simulink model "HevMmReferenceApplication"  (R2021b)
settings: Solver=ode23tb  StartTime=0  StopTime=1800  RelTol=1e-3  EnableMultiTasking=on
model workspace (MAT data in the model file):
  Active_Scenario_Index = 1
  BattChrgMax = -105500
  BattDischrgMax = 211000
  BattTempInit = 25
  Battery.SOC_LUT = [0.01 0.02 0.03 0.04 0.05 0.06 0.07 0.08 0.09 0.1 0.11 0.12 0.13 0.14 0.15 0.16 0.17 0.18 0.19 0.2 0.21 0.22 0.23 0.24 0.25 0.26 0.27 0.28 0.29 0.3 0.31 0.32 0.33 0.34 0.35 0.36 0.37 0.38 0.39 0.4 0.41 0.42 0.43 0.44 0.45 0.46 0.47 0.48 0.49 0.5 0.51 0.52 0.53 0.54 0.55 0.56 0.57 0.58 0.59 0.6 0.61 0.62 0.63 0.64 0.65 0.66 0.67 0.68 0.69 0.7 0.71 0.72 0.73 0.74 0.75 0.76 0.77 0.78 0.79 0.8 0.81 0.82 0.83 0.84 0.85 0.86 0.87 0.88 0.89 0.9 0.91 0.92 0.93 0.94 0.95 0.96 0.97 0.98 0.99 1]
  Battery.Temperature_LUT = [-10 0 25 40]
  Battery.Capacity_LUT = [4.04528301887 4.19622641509 4.8 4.73962264151]
  Battery.Em_LUT = [2.67308083891 2.74411674384 2.80408613071 2.86247711994 2.90851059763 2.94904306488 2.9829846776 3.01467102589 3.04031502638 3.06256828113 3.08180972392 3.09994219643 ... (400 elements, 100x4)]
  Battery.R0_LUT = [0.0569026752707 0.0575506938969 0.0576730924021 0.0575627404981 0.0573787336615 0.0571931123197 0.0568199985482 0.056411926464 0.0561974340667 0.0560805640861 0.0557640899305 0.055275807865 ... (400 elements, 100x4)]
  Battery.R1_LUT = [0.0035 0.0035 0.0035 0.0035 0.0035 0.0035 0.0035 0.0035 0.0035 0.0035 0.0035 0.0035 ... (400 elements, 100x4)]
  Battery.C1_LUT = [5000 5000 5000 5000 5000 5000 5000 5000 5000 5000 5000 5000 ... (400 elements, 100x4)]
  Battery.Mass = 0.047
  Battery.ThermalMass = 44
  Battery.R_bleed = 20
  Battery.h_conv = 5
  Battery.cell_area = 0.0037
  Battery.TempInit = 25
  Battery.SOCInit = 0.75
  Battery.Model = 'panasonic ncr18650bd'
  Battery.DischargeCycle_LUT = [1 5 9 13 17 21 25 29 33 37 41 45 49 53 57 61 65 69 73 77 81 85 89 93 97 101 105 109 113 117 121 125 129 133 137 141 145 149 153 157 161 165 169 173 177 181 185 189 193 197 201 205 209 213 217 221 225 229 233 237 241 245 249 253 257 261 265 269 273 277 281 285 289 293 297 301 305 309 313 317]
  Battery.deltaEm_LUT = [0 -0.363115641304 -0.600096647258 -0.689070000839 -0.76773380251 -0.846397604181 -0.926368385458 -0.992711297521 -1.05704974111 -1.12227693902 -1.19018070587 -1.25808447272 -1.31699459748 -1.35876443799 -1.40168267642 -1.44460091485 -1.48751915327 -1.5304373917 -1.57335563013 -1.62198241593 -1.67232184498 -1.71858340023 -1.76179802551 -1.8050126508 -1.84822727608 -1.8917937136 -1.93575272784 -1.97971174208 -2.02367075632 -2.06762977056 -2.11171979109 -2.15588700406 -2.19980020032 -2.24365853098 -2.28751686164 -2.33137519231 -2.37523352297 -2.41909185363 -2.45982559031 -2.49599372373 -2.53216185715 -2.56832999058 -2.604498124 -2.64066625743 -2.67683439085 -2.71300252428 -2.7491706577 -2.78367585394 -2.81632179346 -2.8483348579 -2.88034792233 -2.91236098677 -2.94437405121 -2.97638711564 -3.00840018008 -3.04041324451 -3.07260346059 -3.10359008254 -3.13082308991 -3.15805609728 -3.18528910464 -3.21252211201 -3.23975511938 -3.26698812675 -3.29422113412 -3.32122400938 -3.3463475604 -3.37152613073 -3.39670470105 -3.42188327138 -3.4470618417 -3.47224041203 -3.49938358795 -3.52900276724 -3.55862194653 -3.58824112582 -3.6178603051 -3.64748858268 -3.67711690909 -3.70674523549]
  Battery.deltaCapacity_LUT = [0 -0.860019120059 -1.71332421702 -2.0819400264 -2.45055583577 -2.81917164515 -3.18778745452 -3.48884924257 -3.7808148236 -4.07278040463 -4.36474598566 -4.6567115667 -4.91000721732 -5.08494410056 -5.2598809838 -5.43481786703 -5.60975475027 -5.78469163351 -5.95962851674 -6.13456539998 -6.30950228322 -6.47026795816 -6.62044510558 -6.77062225299 -6.92079940041 -7.07097654783 -7.22115369524 -7.37133084266 -7.52150799007 -7.67168513749 -7.82230984162 -7.97319825819 -8.12408667477 -8.27497509134 -8.42586350792 -8.57675192449 -8.72764034107 -8.87852875764 -9.01789522921 -9.13717923376 -9.25646323831 -9.37574724285 -9.4950312474 -9.61431525195 -9.73359925649 -9.85288326104 -9.97216726558 -10.0914512701 -10.2059878191 -10.3183039593 -10.4306200996 -10.5429362398 -10.65525238 -10.7675685203 -10.8798846605 -10.9922008008 -11.104516941 -11.2125891929 -11.3075699376 -11.4025506823 -11.4975314271 -11.5925121718 -11.6874929166 -11.7824736613 -11.877454406 -11.9716325175 -12.0588579537 -12.1460833899 -12.2333088261 -12.3205342623 -12.4077596986 -12.4949851348 -12.5890165008 -12.6916254178 -12.7942343349 -12.8968432519 -12.999452169 -13.102061086 -13.2046700031 -13.3072789201]
  Battery.cond_thickness = 0.001
  Battery.thermal_conductivity = 205
  BrkPrsMax = 5000000
  CellType = 1
  ChrgLmt_bpt = [1 1 1 1 1 1 1 1 0.7 0.35 0]
  DischrgLmt_bpt = [0 0.35 0.7 1 1 1 1 1 1 1 1]
  MotMapEff = 0
  MotSpd = [0 1600 3200 4477.56 4800 6400 8000 9600 11200 12800 14400 16000]
  MotTrq = [450 450 450 450 419.771162405 314.828371804 251.862697443 209.885581202 179.901926745 157.414185902 139.923720802 125.931348721]
  Ndiff = 9.04
  Np_Module = 31
  Ns_Module = 24
  NumModules = 4
  OverCellVoltageLimit = 4.19999980927
  RegenBrkCutOff = [0 1]
  RegenBrkSpd_bpt = [5 9]
  Rm = 0.15
  SOC_bpt = [0 10 20 30 40 50 60 70 80 90 100]
  T_eff_bp = [0 32.1428571429 64.2857142857 96.4285714286 128.571428571 160.714285714 192.857142857 225 257.142857143 289.285714286 321.428571429 353.571428571 385.714285714 417.857142857 450]
  TestCase = 1
  UnderCellVoltageLimit = 2.5
  disk_abore = 0.05
  efficiency_table = [86.7  86.7  86.7  86.7  86.7  86.7  86.7  86.7  86.7  86.7  86.7  86.7  86.7  86.7  86.7; 86.7  86.7  86.7  86.7  86.7  86.7  86.7  86.7  86.7  86.7  86.7  86.7  86.7  86.7  86.7; 86.7  86.7  91.8  91.8  91.8  91.8  91.8  91.8  91.8  91.8  89.76  89.76  89.76  89.76  89.76; 86.7  86.7  93.84  93.84  93.84  93.84  93.84  93.84  93.84  93.84  93.84  91.8  91.8  91.8  91.8; 86.7  86.7  93.84  93.84  94.86  94.86  94.86  94.86  93.84  93.84  93.84  91.8  91.8  91.8  91.8; 86.7  86.7  94.86  95.88  95.88  95.88  95.88  95.88  95.88  95.88  95.88  95.88  95.88  95.88  95.88; 86.7  86.7  94.86  95.88  95.88  96.9  96.9  96.9  96.9  96.9  96.9  96.9  96.9  96.9  96.9; 86.7  86.7  94.86  95.88  95.88  96.9  96.9  96.9  96.9  96.9  96.9  96.9  96.9  96.9  96.9; 86.7  86.7  94.86  95.88  96.9  96.9  96.9  96.9  96.9  96.9  96.9  96.9  96.9  96.9  96.9; 86.7  86.7  94.86  95.88  96.9  96.9  96.9  96.9  96.9  96.9  96.9  96.9  96.9  96.9  96.9; 86.7  86.7  94.86  95.88  95.88  95.88  95.88  95.88  95.88  95.88  95.88  95.88  95.88  95.88  95.88; 86.7  86.7  91.8  93.84  94.86  94.86  94.86  94.86  94.86  94.86  94.86  94.86  94.86  94.86  94.86]
  mu_kinetic = 0.35
  num_pads = 2
  ts = 0.1
  w_eff_bp = [0 1600 3200 4477.56 4800 6400 8000 9600 11200 12800 14400 16000]
undefined symbols (not defined in the file or in its folder): sigbuilder_block, SRE
libraries: autolibsharedcommon x4, autolibshared x3, simulink x1, slpidlib x1
(part 1 of 2)
settings Model: DataDictionary=HevMmReferenceApplication.sldd  ModifiedByFormat=The MathWorks, Inc.  SimulationMode=accelerator  PauseTimes=23.46  Creator=The MathWorks, Inc.  LastModifiedBy=The MathWorks, Inc.
settings SolverCC: SolverJacobianMethodControl=FullPerturbation  ZeroCrossAlgorithm=Adaptive  AlgebraicLoopSolver=TrustRegion  MinimalZcImpactIntegration=on
settings DataIOCC: DSMLogging=off  ReturnWorkspaceOutputs=off
settings DebuggingCC: UnderspecifiedInitializationDetection=Classic  MergeDetectMultiDrivingBlocksExec=none  MaskedZcDiagnostic=none  IgnoredZcDiagnostic=none  ParameterPrecisionLossMsg=none  ModelReferenceExtraNoncontSigs=none  PregeneratedLibrarySubsystemCodeDiagnostic=none  SFMachineParentedDataDiag=warning  ArithmeticOperatorsInVariantConditions=warning
settings ModelReferenceCC: UpdateModelReferenceTargets=IfOutOfDate  ModelReferenceMinAlgLoopOccurrences=on  PropagateSignalLabelsOutOfModel=off
settings SFSimCC: SimUseLocalCustomCode=off
settings RTWCC: RTWUseLocalCustomCode=off
settings CodeAppCC: StateflowObjectComments=on
settings GRTTargetCC: TargetLangStandard=C89/C90 (ANSI)
settings ConfigComp: CovMetricSettings=dsw  CovSaveCumulativeToWorkspaceVar=on  CovSaveSingleToWorkspaceVar=on  CovExternalEMLEnable=off

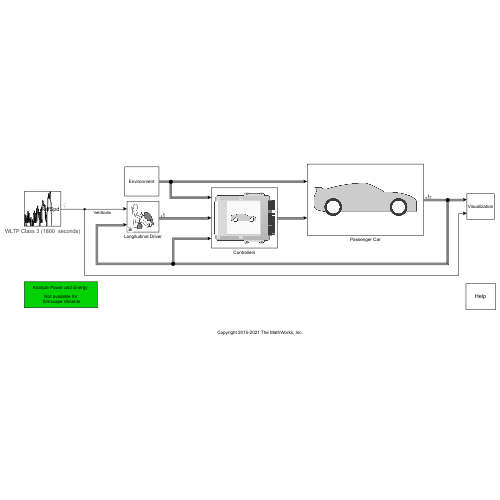
[thumbnail: Simulink's stored preview of the top-level diagram]
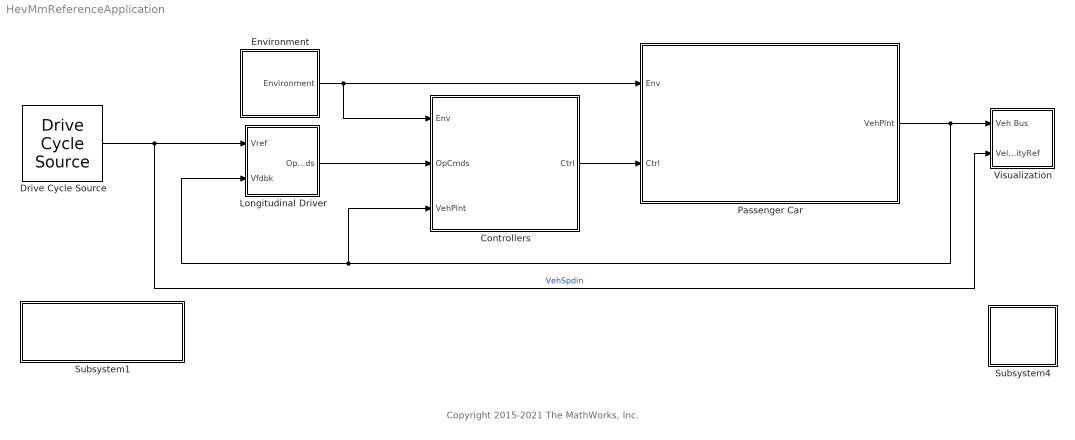
== system HevMmReferenceApplication ==
  note: Copyright 2015-2021 The MathWorks, Inc.
  Controllers : Subsystem
      mask Display: image('SystemControllers.png', 'center')
  Drive Cycle Source : autolibshared/Drive Cycle Source  cycleVar=WLTP Class 3  fileVar=L:\Bauto\matlab\test\toolbox\shared\autoblks\scenario\adac.txt  tfinal="1800  seconds"  cycleRepeat=off  outAccPort=off  outGearPort=off  gearList=No gear data  t_wot1=1  xdot_woto=0  xdot_wot1=10  t_wot2=199  xdot_wot2=0  t_wotend=200  srcUnit=m/s  outUnit=m/s  srcAccUnit=m/s/s  outAccUnit=m/s^2  dt=0  aMode=1  faultOption=off  velBnd=2  velBndUnit=mph  inUnit=m/s  timeBnd=1  failOption=off  stopSim=off  maxFaultCnt=10  maxFaultTime=2  maxTotFaultTime=15  traceOption=off  dtTrace=1  traceWindow=10  lastDCname=WLTP Class 3  lastOutUnit=mph  lastDT=0  lastTB=1  lastSB=2  forceCalcBound=off
      settings: SourceProductBaseCode=PW,DR,MT,UV,VE
  Environment : Subsystem
      mask Display: disp(getString(message('autoblks:autoblkVehMask:environ')))
  Longitudinal Driver : Subsystem  Variant=on  VariantControlMode=label  VariantControl=Variant1  LabelModeActiveChoice=2
      mask Display:
      | if strcmp('1',get_param(gcb,'ActiveVariant'))
      |     disp('Open Loop')
      | else
      |     image('LongitudinalDriver.png','center');
      | end
  Passenger Car : Subsystem
      mask Display: image('PassengerVehicle.png', 'center')
  Subsystem1 : Subsystem
      settings: OpenFcn=edit GenerateEnergyReport
      mask Display: disp(getString(message('autoblks:autoblkVehMask:powAndEne')))
  Subsystem4 : Subsystem
      settings: OpenFcn=helpview([docroot,'/toolbox/autoblks/helptargets.map'], 'hybrid_refapp')
      mask Display: disp(getString(message('autoblks:autoblkVehMask:help')))
  Visualization : Subsystem
      mask Display: disp(getString(message('autoblks:autoblkVehMask:visual')))
  wires:
  Longitudinal Driver/1(" OpCmds") -> Controllers/2(OpCmds)
  Drive Cycle Source/1 -> Longitudinal Driver/1("Vref "), Visualization/2(VelocityRef)  "VehSpdin"
  Environment/1(Environment) -> Passenger Car/1(Env), Controllers/1(Env)
  Controllers/1(Ctrl) -> Passenger Car/2(Ctrl)
  Passenger Car/1(VehPlnt) -> Longitudinal Driver/2("Vfdbk "), Controllers/3(VehPlnt), Visualization/1(Veh Bus)

== system HevMmReferenceApplication/Controllers ==
  Env : Inport
  OpCmds : Inport  Port=2
  VehPlnt : Inport  Port=3
  Bus Creator : BusCreator  Inputs=2
  PCM Input : Subsystem
  PCM Output : Subsystem
  Powertrain Control Module (PCM) : Subsystem
  Ctrl : Outport  VectorParamsAs1DForOutWhenUnconnected=off
  wires:
  PCM Output/1(EngCtrl) -> [EngCtrl]
  Bus Creator/1 -> Ctrl/1
  [EngCtrl] -> Bus Creator/1
  [PtCtrl] -> Bus Creator/2
  Env/1 -> [Environment]
  [OpCmds] -> PCM Input/4(OpCmds)
  VehPlnt/1 -> [VehPlnt]
  OpCmds/1 -> [OpCmds]
  [PtCtrl] -> PCM Input/1(PtCtrl)
  [Environment] -> PCM Input/2(Env)
  [VehPlnt] -> PCM Input/3(VehPlnt)
  PCM Output/2(PtCtrl) -> [PtCtrl]
  PCM Input/1(TrqCmd) -> Powertrain Control Module (PCM)/1(TrqCmd)
  PCM Input/2(EngSpd) -> Powertrain Control Module (PCM)/2(EngSpd)
  PCM Input/3(Map) -> Powertrain Control Module (PCM)/3(Map)
  PCM Input/4(Mat) -> Powertrain Control Module (PCM)/4(Mat)
  PCM Input/5(ThrPosPct) -> Powertrain Control Module (PCM)/5(ThrPosPct)
  PCM Input/6(WgAreaPct) -> Powertrain Control Module (PCM)/6(WgAreaPct)
  PCM Input/7(IntkCamPhase) -> Powertrain Control Module (PCM)/7(IntkCamPhase)
  PCM Input/8(ExhCamPhase) -> Powertrain Control Module (PCM)/8(ExhCamPhase)
  PCM Input/9(TurboRackPos) -> Powertrain Control Module (PCM)/9(TurboRackPos)
  PCM Input/10(EgrVlvAreaPct) -> Powertrain Control Module (PCM)/10(EgrVlvAreaPct)
  PCM Input/11(VarCompRatioPos) -> Powertrain Control Module (PCM)/11(VarCompRatioPos)
  PCM Input/12(IntkVlvLift) -> Powertrain Control Module (PCM)/12(IntkVlvLift)
  PCM Input/13(VarIntkRunLen) -> Powertrain Control Module (PCM)/13(VarIntkRunLen)
  PCM Input/14(Afr) -> Powertrain Control Module (PCM)/14(Afr)
  PCM Input/15(IntkSwirlVlvPos) -> Powertrain Control Module (PCM)/15(IntkSwirlVlvPos)
  PCM Input/16(TurboSpd) -> Powertrain Control Module (PCM)/16(TurboSpd)
  PCM Input/17(AmbPrs) -> Powertrain Control Module (PCM)/17(AmbPrs)
  PCM Input/18(AccCmd) -> Powertrain Control Module (PCM)/18(AccCmd)
  PCM Input/19(DecCmd) -> Powertrain Control Module (PCM)/19(DecCmd)
  PCM Input/25(VehSpdFdbk) -> Powertrain Control Module (PCM)/25(VehSpdFdbk)
  PCM Input/26(EngSpdFdbk) -> Powertrain Control Module (PCM)/26(EngSpdFdbk)
  PCM Input/27(EngCltchState) -> Powertrain Control Module (PCM)/27(EngCltchState)
  PCM Input/28(BattSoc) -> Powertrain Control Module (PCM)/28(BattSoc)
  PCM Input/29(BattPwr) -> Powertrain Control Module (PCM)/29(BattPwr)
  PCM Input/30(BattCrnt) -> Powertrain Control Module (PCM)/30(BattCrnt)
  PCM Input/31(EngCltchOutSpd) -> Powertrain Control Module (PCM)/31(EngCltchOutSpd)
  PCM Input/32(MotSpd) -> Powertrain Control Module (PCM)/32(MotSpd)
  PCM Input/33(GenPwrElec) -> Powertrain Control Module (PCM)/33(GenPwrElec)
  PCM Input/34(GenPwrMech) -> Powertrain Control Module (PCM)/34(GenPwrMech)
  PCM Input/20(IgSw) -> Powertrain Control Module (PCM)/20(IgSw)
  PCM Input/22(Ect) -> Powertrain Control Module (PCM)/22(Ect)
  PCM Input/23(EgrDeltaPrs) -> Powertrain Control Module (PCM)/23(EgrVlvDeltaPrs)
  PCM Input/24(EgrInTemp) -> Powertrain Control Module (PCM)/24(EgrVlvInTemp)
  PCM Input/21(Iat) -> Powertrain Control Module (PCM)/21(Iat)
  Powertrain Control Module (PCM)/1(ThrPosPctCmd) -> PCM Output/1(ThrPosPctCmd)
  Powertrain Control Module (PCM)/2(WgAreaPctCmd) -> PCM Output/2(WgAreaPctCmd)
  Powertrain Control Module (PCM)/3(InjPw) -> PCM Output/3(InjPw)
  Powertrain Control Module (PCM)/4(FuelMainSoi) -> PCM Output/4(FuelMainSoi)
  Powertrain Control Module (PCM)/5(SpdAdv) -> PCM Output/5(SpkAdv)
  Powertrain Control Module (PCM)/6(IntkCamPhaseCmd) -> PCM Output/6(IntkCamPhaseCmd)
  Powertrain Control Module (PCM)/7(ExhCamPhaseCmd) -> PCM Output/7(ExhCamPhaseCmd)
  Powertrain Control Module (PCM)/8(TurboRackPosCmd) -> PCM Output/8(TurboRackPosCmd)
  Powertrain Control Module (PCM)/9(EgrVlvAreaPctCmd) -> PCM Output/9(EgrVlvAreaPctCmd)
  Powertrain Control Module (PCM)/10(VarCompRatioPosCmd) -> PCM Output/10(VarCompRatioPosCmd)
  Powertrain Control Module (PCM)/11(IntkVlvLiftCmd) -> PCM Output/11(IntkVlvLiftCmd)
  Powertrain Control Module (PCM)/12(VarIntkRunLenCmd) -> PCM Output/12(VarIntkRunLenCmd)
  Powertrain Control Module (PCM)/13(ClsdLpFuelMult) -> PCM Output/13(ClsdLpFuelMult)
  Powertrain Control Module (PCM)/14(IntkSwirlVlvPosCmd) -> PCM Output/14(IntkSwirlVlvPosCmd)
  Powertrain Control Module (PCM)/15(TrqCmdISC) -> PCM Output/15(TrqCmdISC)
  Powertrain Control Module (PCM)/16(LoadCmd) -> PCM Output/16(LoadCmd)
  Powertrain Control Module (PCM)/17(EstIntkPortFlw) -> PCM Output/17(EstIntkPortFlw)
  Powertrain Control Module (PCM)/18(EngCltchCmd) -> PCM Output/18(EngCltchCmd)
  Powertrain Control Module (PCM)/19(EngTrqCmd) -> PCM Output/19(EngineTrqCmd)
  Powertrain Control Module (PCM)/20(GenTrqCmd) -> PCM Output/20(GenTrqCmd)
  Powertrain Control Module (PCM)/21(MotTrqCmd) -> PCM Output/21(MotTrqCmd)
  Powertrain Control Module (PCM)/22(BrakeCmd) -> PCM Output/22(BrakeCmd)
  PCM Input/35(BMS_Sensors) -> Powertrain Control Module (PCM)/35(BMS_Sensors)
  Powertrain Control Module (PCM)/23(BMS_Info) -> PCM Output/23(BMS_Info)
  Powertrain Control Module (PCM)/24(BMS_Cmd) -> PCM Output/24(BMS_Cmd)

== system HevMmReferenceApplication/Environment ==
  Bus Creator : BusCreator  Inputs=4
  Bus Creator3 : BusCreator  Inputs=3
  Bus Creator4 : BusCreator  Inputs=2
  Bus Creator5 : BusCreator  Inputs=2
  Constant2 : Constant  Value=0
  Constant3 : Constant  Value=0
  Constant6 : Constant  Value=300
  Constant7 : Constant  Value=101325
  Ground{,1..3} (4 alike) : Ground
  Environment : Outport  VectorParamsAs1DForOutWhenUnconnected=off
  wires:
  Ground2/1 -> Bus Creator5/1  "lam_mu_x"
  Ground3/1 -> Bus Creator5/2  "lam_mu_y"
  Bus Creator5/1 -> Bus Creator4/2  "Ground_mu"
  Bus Creator4/1 -> Bus Creator/3  "Ground"
  Bus Creator3/1 -> Bus Creator/4  "Wind"
  Constant3/1 -> Bus Creator3/1  "wind_x"
  Ground/1 -> Bus Creator3/2  "wind_y"
  Ground1/1 -> Bus Creator3/3  "wind_z"
  Constant6/1 -> Bus Creator/1  "Temp"
  Constant2/1 -> Bus Creator4/1  "Grade"
  Bus Creator/1 -> Environment/1  "Environment"
  Constant7/1 -> Bus Creator/2  "Baro"

== system HevMmReferenceApplication/Longitudinal Driver ==
  note: To switch variants, right-click on this subsystem (from one level above) and chose:
      | Variant, Active choice, <your selection>
  "Vref " : Inport
  "Vfdbk " : Inport  Port=2
  Longitudinal Driver : Subsystem  VariantControl=0
      mask Display: image('LongitudinalDriver.png', 'center')
  Open Loop : Subsystem  VariantControl=1
      mask Display: disp('Open Loop')
  PID : Subsystem  TreatAsAtomicUnit=on  VariantControl=2
  " OpCmds" : Outport  VectorParamsAs1DForOutWhenUnconnected=off

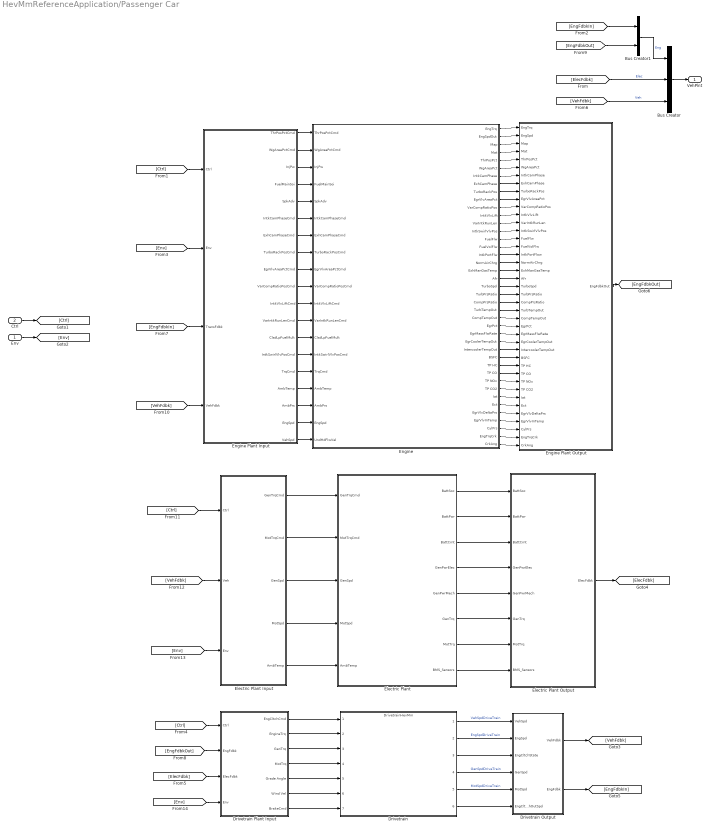
== system HevMmReferenceApplication/Passenger Car ==
  Env : Inport
  Ctrl : Inport  Port=2
  Bus Creator : BusCreator  Inputs=3
  Bus Creator1 : BusCreator  Inputs=2
  Drivetrain : ModelReference  ModelNameDialog=DrivetrainHevMm.slx  SimulationMode=Normal  ModelReferenceVersion=5.24
  Drivetrain Output : Subsystem
  Drivetrain Plant Input : Subsystem
  Electric Plant : Subsystem
  Electric Plant Input : Subsystem
  Electric Plant Output : Subsystem
  Engine : Subsystem  Variant=on  VariantControlMode=label  LabelModeActiveChoice=SiMappedEngine
  Engine Plant Input : Subsystem
  Engine Plant Output : Subsystem
  VehPlnt : Outport  VectorParamsAs1DForOutWhenUnconnected=off
  wires:
  Ctrl/1 -> [Ctrl]
  Env/1 -> [Env]
  [Ctrl] -> Drivetrain Plant Input/1(Ctrl)
  [EngFdbkOut] -> Drivetrain Plant Input/2(EngFdbk)
  Engine Plant Output/1(EngFdbkOut) -> [EngFdbkOut]
  [Ctrl] -> Engine Plant Input/1(Ctrl)
  [Env] -> Engine Plant Input/2(Env)
  [EngFdbkIn] -> Engine Plant Input/3(TransFdbk)
  [VehFdbk] -> Engine Plant Input/4(VehFdbk)
  Bus Creator/1 -> VehPlnt/1
  [EngFdbkIn] -> Bus Creator1/1
  [VehFdbk] -> Bus Creator/3  "Veh"
  Bus Creator1/1 -> Bus Creator/1  "Eng"
  [EngFdbkOut] -> Bus Creator1/2
  Drivetrain Output/1(VehFdbk) -> [VehFdbk]
  Drivetrain Output/2(EngFdbk) -> [EngFdbkIn]
  Drivetrain/1 -> Drivetrain Output/1(VehSpd)  "VehSpdDriveTrain"
  Drivetrain/2 -> Drivetrain Output/2("EngSpd ")  "EngSpdDriveTrain"
  Drivetrain/3 -> Drivetrain Output/3(EngCltchState)
  Drivetrain/4 -> Drivetrain Output/4(GenSpd)  "GenSpdDriveTrain"
  Electric Plant Output/1(ElecFdbk) -> [ElecFdbk]
  [ElecFdbk] -> Bus Creator/2  "Elec"
  [Ctrl] -> Electric Plant Input/1(Ctrl)
  [ElecFdbk] -> Drivetrain Plant Input/3(ElecFdbk)
  Drivetrain Plant Input/4(MotTrq) -> Drivetrain/4
  Drivetrain Plant Input/3(GenTrq) -> Drivetrain/3
  Drivetrain Plant Input/1(EngCltchCmd) -> Drivetrain/1
  Drivetrain Plant Input/2(EngineTrq) -> Drivetrain/2
  Drivetrain Plant Input/7(BrakeCmd) -> Drivetrain/7
  Drivetrain/5 -> Drivetrain Output/5(MotSpd)  "MotSpdDriveTrain"
  [VehFdbk] -> Electric Plant Input/2(Veh)
  Drivetrain/6 -> Drivetrain Output/6(EngCltchOutSpd)
  Electric Plant Input/1(GenTrqCmd) -> Electric Plant/1(GenTrqCmd)
  Electric Plant Input/2(MotTrqCmd) -> Electric Plant/2(MotTrqCmd)
  Electric Plant Input/3(GenSpd) -> Electric Plant/3(GenSpd)
  Electric Plant Input/4(MotSpd) -> Electric Plant/4(MotSpd)
  Electric Plant/1(BattSoc) -> Electric Plant Output/1(BattSoc)
  Electric Plant/2(BattPwr) -> Electric Plant Output/2(BattPwr)
  Electric Plant/3(BattCrnt) -> Electric Plant Output/3(BattCrnt)
  Electric Plant/4(GenPwrElec) -> Electric Plant Output/4(GenPwrElec)
  Electric Plant/5(GenPwrMech) -> Electric Plant Output/5(GenPwrMech)
  Electric Plant/6(GenTrq) -> Electric Plant Output/6(GenTrq)
  Electric Plant/7(MotTrq) -> Electric Plant Output/7(MotTrq)
  [Env] -> Electric Plant Input/3(Env)
  Electric Plant Input/5(AmbTemp) -> Electric Plant/5(AmbTemp)
  [Env] -> Drivetrain Plant Input/4(Env)
  Drivetrain Plant Input/5(Grade Angle) -> Drivetrain/5
  Drivetrain Plant Input/6(Wind Vel) -> Drivetrain/6
  Engine Plant Input/19(VehSpd) -> Engine/19(UndHdFlwVel)
  Engine Plant Input/16(AmbTemp) -> Engine/16(AmbTemp)
  Engine Plant Input/13(ClsdLpFuelMult) -> Engine/13(ClsdLpFuelMult)
  Engine Plant Input/12(VarIntkRunLenCmd) -> Engine/12(VarIntkRunLenCmd)
  Engine Plant Input/14(IntkSwirlVlvPosCmd) -> Engine/14(IntkSwirlVlvPosCmd)
  Engine Plant Input/9(EgrVlvAreaPctCmd) -> Engine/9(EgrVlvAreaPctCmd)
  Engine Plant Input/5(SpkAdv) -> Engine/5(SpkAdv)
  Engine Plant Input/4(FuelMainSoi) -> Engine/4(FuelMainSoi)
  Engine Plant Input/18(EngSpd) -> Engine/18(EngSpd)
  Engine Plant Input/10(VarCompRatioPosCmd) -> Engine/10(VarCompRatioPosCmd)
  Engine Plant Input/7(ExhCamPhaseCmd) -> Engine/7(ExhCamPhaseCmd)
  Engine Plant Input/6(IntkCamPhaseCmd) -> Engine/6(IntkCamPhaseCmd)
  Engine Plant Input/2(WgAreaPctCmd) -> Engine/2(WgAreaPctCmd)
  Engine Plant Input/8(TurboRackPosCmd) -> Engine/8(TurboRackPosCmd)
  Engine Plant Input/15(TrqCmd) -> Engine/15(TrqCmd)
  Engine Plant Input/3(InjPw) -> Engine/3(InjPw)
  Engine Plant Input/17(AmbPrs) -> Engine/17(AmbPrs)
  Engine Plant Input/11(IntkVlvLiftCmd) -> Engine/11(IntkVlvLiftCmd)
  Engine Plant Input/1(ThrPosPctCmd) -> Engine/1(ThrPosPctCmd)
  Engine/17(IntkPortFlw) -> Engine Plant Output/17(IntkPortFlow)
  Engine/16(FuelVolFlw) -> Engine Plant Output/16(FuelVolFlw)
  Engine/18(NormAirChrg) -> Engine Plant Output/18(NormAirChrg)
  Engine/15(FuelFlw) -> Engine Plant Output/15(FuelFlw)
  Engine/19(ExhManGasTemp) -> Engine Plant Output/19(ExhManGasTemp)
  Engine/14(IntkSwirlVlvPos) -> Engine Plant Output/14(IntkSwirlVlvPos)
  Engine/20(Afr) -> Engine Plant Output/20(Afr)
  Engine/21(TurboSpd) -> Engine Plant Output/21(TurboSpd)
  Engine/13(VarIntkRunLen) -> Engine Plant Output/13(VarIntkRunLen)
  Engine/22(TurbPrsRatio) -> Engine Plant Output/22(TurbPrsRatio)
  Engine/12(IntkVlvLift) -> Engine Plant Output/12(IntkVlvLift)
  Engine/23(CompPrsRatio) -> Engine Plant Output/23(CompPrsRatio)
  Engine/11(VarCompRatioPos) -> Engine Plant Output/11(VarCompRatioPos)
  Engine/24(TurbTempOut) -> Engine Plant Output/24(TurbTempOut)
  Engine/10(EgrVlvAreaPct) -> Engine Plant Output/10(EgrVlvAreaPct)
  Engine/25(CompTempOut) -> Engine Plant Output/25(CompTempOut)
  Engine/9(TurboRackPos) -> Engine Plant Output/9(TurboRackPos)
  Engine/26(EgrPct) -> Engine Plant Output/26(EgrPct)
  Engine/8(ExhCamPhase) -> Engine Plant Output/8(ExhCamPhase)
  Engine/27(EgrMassFlwRate) -> Engine Plant Output/27(EgrMassFlwRate)
  Engine/7(IntkCamPhase) -> Engine Plant Output/7(IntkCamPhase)
  Engine/28(EgrCoolerTempOut) -> Engine Plant Output/28(EgrCoolerTempOut)
  Engine/6(WgAreaPct) -> Engine Plant Output/6(WgAreaPct)
  Engine/29(IntercoolerTempOut) -> Engine Plant Output/29(IntercoolerTempOut)
  Engine/5(ThrPosPct) -> Engine Plant Output/5(ThrPosPct)
  Engine/30(BSFC) -> Engine Plant Output/30(BSFC)
  Engine/4(Mat) -> Engine Plant Output/4(Mat)
  Engine/31(TP HC) -> Engine Plant Output/31(TP HC)
  Engine/3(Map) -> Engine Plant Output/3(Map)
  Engine/32(TP CO) -> Engine Plant Output/32(TP CO)
  Engine/2(EngSpdOut) -> Engine Plant Output/2(EngSpd)
  Engine/33(TP NOx) -> Engine Plant Output/33(TP NOx)
  Engine/1(EngTrq) -> Engine Plant Output/1(EngTrq)
  Engine/34(TP CO2) -> Engine Plant Output/34(TP CO2)
  Engine/35(Iat) -> Engine Plant Output/35(Iat)
  Engine/36(Ect) -> Engine Plant Output/36(Ect)
  Engine/37(EgrVlvDeltaPrs) -> Engine Plant Output/37(EgrVlvDeltaPrs)
  Engine/38(EgrVlvInTemp) -> Engine Plant Output/38(EgrVlvInTemp)
  Engine/39(CylPrs) -> Engine Plant Output/39(CylPrs)
  Engine/40(EngTrqCrk) -> Engine Plant Output/40(EngTrqCrk)
  Engine/41(CrkAng) -> Engine Plant Output/41(CrkAng)
  Electric Plant/8(BMS_Sensors) -> Electric Plant Output/8(BMS_Sensors)

== system HevMmReferenceApplication/Subsystem1 ==

== system HevMmReferenceApplication/Subsystem4 ==

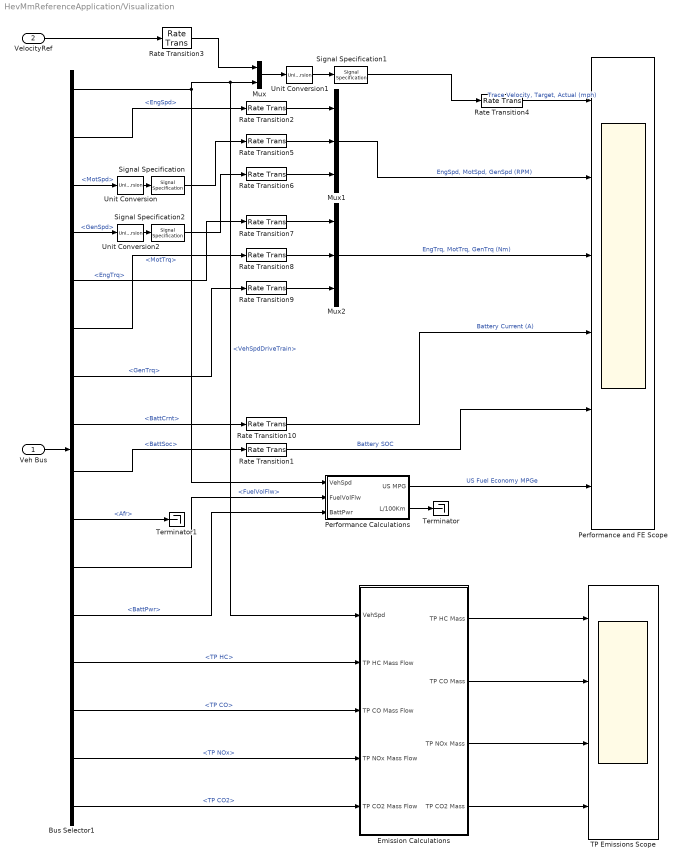
== system HevMmReferenceApplication/Visualization ==
  Veh Bus : Inport
  VelocityRef : Inport  Port=2
  Bus Selector1 : BusSelector  OutputSignals=Veh.VehSpdDriveTrain,Eng.EngFdbkOut.EngSpd,Veh.MotSpd,Veh.GenSpd,Eng.EngFdbkOut.EngTrq,Elec.MotTrq,Elec.GenTrq,Elec.BattCrnt,Elec.BattSoc,Eng.EngFdbkOut.Afr,Eng.EngFdbkOut.FuelVolFlw,Elec.BattPwr,Eng.EngFdbkOut.TP HC,Eng.EngFdbkOut.TP CO,Eng.EngFdbkOut.TP NOx,Eng.EngFdbkOut.TP CO2
  Emission Calculations : Subsystem
  Mux : Mux  Inputs=2
  Mux1 : Mux  Inputs=3
  Mux2 : Mux  Inputs=3
  Performance Calculations : Subsystem
  Performance and FE Scope : Scope  NumInputPorts=6
  Rate Transition{1..10} (10 alike) : RateTransition  Deterministic=off
  Signal Specification : SignalSpecification  Unit=rpm
  Signal Specification1 : SignalSpecification  Unit=mph
  Signal Specification2 : SignalSpecification  Unit=rpm
  TP Emissions Scope : Scope  NumInputPorts=4
  Terminator : Terminator
  Terminator1 : Terminator
  Unit Conversion : UnitConversion
  Unit Conversion1 : UnitConversion
  Unit Conversion2 : UnitConversion
  wires:
  Veh Bus/1 -> Bus Selector1/1
  Bus Selector1/1 -> Mux/2, Emission Calculations/1(VehSpd), Performance Calculations/1(VehSpd)  "<VehSpdDriveTrain>"
  Bus Selector1/2 -> Rate Transition2/1  "<EngSpd>"
  Mux/1 -> Unit Conversion1/1
  Bus Selector1/11 -> Performance Calculations/2(FuelVolFlw)  "<FuelVolFlw>"
  Performance Calculations/1(US MPG) -> Performance and FE Scope/6  "US Fuel Economy MPGe"
  Performance Calculations/2(L/100Km) -> Terminator/1
  Bus Selector1/10 -> Terminator1/1  "<Afr>"
  Signal Specification1/1 -> Rate Transition4/1
  VelocityRef/1 -> Rate Transition3/1
  Bus Selector1/9 -> Rate Transition1/1  "<BattSoc>"
  Bus Selector1/13 -> Emission Calculations/2(TP HC Mass Flow)  "<TP HC>"
  Bus Selector1/14 -> Emission Calculations/3(TP CO Mass Flow)  "<TP CO>"
  Bus Selector1/15 -> Emission Calculations/4(TP NOx Mass Flow)  "<TP NOx>"
  Emission Calculations/1(TP HC Mass) -> TP Emissions Scope/1
  Emission Calculations/2(TP CO Mass) -> TP Emissions Scope/2
  Emission Calculations/3(TP NOx Mass) -> TP Emissions Scope/3
  Bus Selector1/16 -> Emission Calculations/5(TP CO2 Mass Flow)  "<TP CO2>"
  Emission Calculations/4(TP CO2 Mass) -> TP Emissions Scope/4
  Rate Transition3/1 -> Mux/1
  Rate Transition1/1 -> Performance and FE Scope/5  "Battery SOC"
  Mux1/1 -> Performance and FE Scope/2  "EngSpd, MotSpd, GenSpd (RPM)"
  Rate Transition4/1 -> Performance and FE Scope/1  "Trace Velocity, Target, Actual (mph)"
  Bus Selector1/12 -> Performance Calculations/3(BattPwr)  "<BattPwr>"
  Bus Selector1/3 -> Unit Conversion/1  "<MotSpd>"
  Bus Selector1/4 -> Unit Conversion2/1  "<GenSpd>"
  Rate Transition2/1 -> Mux1/1
  Rate Transition5/1 -> Mux1/2
  Rate Transition6/1 -> Mux1/3
  Rate Transition9/1 -> Mux2/3
  Rate Transition8/1 -> Mux2/2
  Rate Transition7/1 -> Mux2/1
  Mux2/1 -> Performance and FE Scope/3  "EngTrq, MotTrq, GenTrq (Nm)"
  Bus Selector1/5 -> Rate Transition7/1  "<EngTrq>"
  Bus Selector1/6 -> Rate Transition8/1  "<MotTrq>"
  Bus Selector1/7 -> Rate Transition9/1  "<GenTrq>"
  Bus Selector1/8 -> Rate Transition10/1  "<BattCrnt>"
  Rate Transition10/1 -> Performance and FE Scope/4  "Battery Current (A)"
  Signal Specification/1 -> Rate Transition5/1
  Signal Specification2/1 -> Rate Transition6/1
  Unit Conversion/1 -> Signal Specification/1
  Unit Conversion1/1 -> Signal Specification1/1
  Unit Conversion2/1 -> Signal Specification2/1

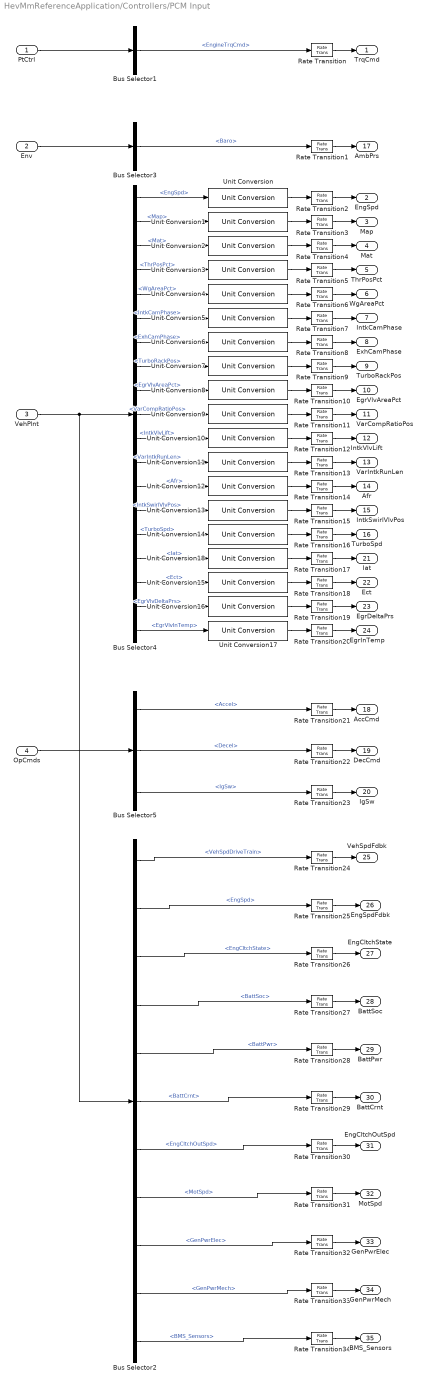
== system HevMmReferenceApplication/Controllers/PCM Input ==
  PtCtrl : Inport
  Env : Inport  Port=2
  VehPlnt : Inport  Port=3
  OpCmds : Inport  Port=4
  Bus Selector1 : BusSelector  OutputSignals=EngineTrqCmd
  Bus Selector2 : BusSelector  OutputSignals=Veh.VehSpdDriveTrain,Eng.EngFdbk.EngSpd,Veh.EngCltchState,Elec.BattSoc,Elec.BattPwr,Elec.BattCrnt,Veh.EngCltchOutSpd,Veh.MotSpd,Elec.GenPwrElec,Elec.GenPwrMech,Elec.BMS_Sensors
  Bus Selector3 : BusSelector  OutputSignals=Baro
  Bus Selector4 : BusSelector  OutputSignals=Eng.EngFdbkOut.EngSpd,Eng.EngFdbkOut.Map,Eng.EngFdbkOut.Mat,Eng.EngFdbkOut.ThrPosPct,Eng.EngFdbkOut.WgAreaPct,Eng.EngFdbkOut.IntkCamPhase,Eng.EngFdbkOut.ExhCamPhase,Eng.EngFdbkOut.TurboRackPos,Eng.EngFdbkOut.EgrVlvAreaPct,Eng.EngFdbkOut.VarCompRatioPos,Eng.EngFdbkOut.IntkVlvLift,Eng.EngFdbkOut.VarIntkRunLen,Eng.EngFdbkOut.Afr,Eng.EngFdbkOut.IntkSwirlVlvPos,Eng.EngFdbkOut.TurboSpd,Eng.EngFdbkOut.Iat,Eng.EngFdbkOut.Ect,Eng.EngFdbkOut.EgrVlvDeltaPrs,Eng.EngFdbkOut.EgrVlvInTemp
  Bus Selector5 : BusSelector  OutputSignals=Info.Accel,Info.Decel,IgSw
  Rate Transition{,1..20,23..34} (33 alike) : RateTransition
  Rate Transition21 : RateTransition  OutPortSampleTimeOpt=Inherit
  Rate Transition22 : RateTransition  OutPortSampleTimeOpt=Inherit
  Unit Conversion{,1..18} (19 alike) : UnitConversion
  TrqCmd : Outport  VectorParamsAs1DForOutWhenUnconnected=off
  EngSpd : Outport  Port=2  VectorParamsAs1DForOutWhenUnconnected=off
  Map : Outport  Port=3  VectorParamsAs1DForOutWhenUnconnected=off
  Mat : Outport  Port=4  VectorParamsAs1DForOutWhenUnconnected=off
  ThrPosPct : Outport  Port=5  VectorParamsAs1DForOutWhenUnconnected=off
  WgAreaPct : Outport  Port=6  VectorParamsAs1DForOutWhenUnconnected=off
  IntkCamPhase : Outport  Port=7  VectorParamsAs1DForOutWhenUnconnected=off
  ExhCamPhase : Outport  Port=8  VectorParamsAs1DForOutWhenUnconnected=off
  TurboRackPos : Outport  Port=9  VectorParamsAs1DForOutWhenUnconnected=off
  EgrVlvAreaPct : Outport  Port=10  VectorParamsAs1DForOutWhenUnconnected=off
  VarCompRatioPos : Outport  Port=11  VectorParamsAs1DForOutWhenUnconnected=off
  IntkVlvLift : Outport  Port=12  VectorParamsAs1DForOutWhenUnconnected=off
  VarIntkRunLen : Outport  Port=13  VectorParamsAs1DForOutWhenUnconnected=off
  Afr : Outport  Port=14  VectorParamsAs1DForOutWhenUnconnected=off
  IntkSwirlVlvPos : Outport  Port=15  VectorParamsAs1DForOutWhenUnconnected=off
  TurboSpd : Outport  Port=16  VectorParamsAs1DForOutWhenUnconnected=off
  AmbPrs : Outport  Port=17  VectorParamsAs1DForOutWhenUnconnected=off
  AccCmd : Outport  Port=18  VectorParamsAs1DForOutWhenUnconnected=off
  DecCmd : Outport  Port=19  VectorParamsAs1DForOutWhenUnconnected=off
  IgSw : Outport  Port=20  VectorParamsAs1DForOutWhenUnconnected=off
  Iat : Outport  Port=21  VectorParamsAs1DForOutWhenUnconnected=off
  Ect : Outport  Port=22  VectorParamsAs1DForOutWhenUnconnected=off
  EgrDeltaPrs : Outport  Port=23  VectorParamsAs1DForOutWhenUnconnected=off
  EgrInTemp : Outport  Port=24  VectorParamsAs1DForOutWhenUnconnected=off
  VehSpdFdbk : Outport  Port=25  VectorParamsAs1DForOutWhenUnconnected=off
  EngSpdFdbk : Outport  Port=26  VectorParamsAs1DForOutWhenUnconnected=off
  EngCltchState : Outport  Port=27  VectorParamsAs1DForOutWhenUnconnected=off
  BattSoc : Outport  Port=28  VectorParamsAs1DForOutWhenUnconnected=off
  BattPwr : Outport  Port=29  VectorParamsAs1DForOutWhenUnconnected=off
  BattCrnt : Outport  Port=30  VectorParamsAs1DForOutWhenUnconnected=off
  EngCltchOutSpd : Outport  Port=31  VectorParamsAs1DForOutWhenUnconnected=off
  MotSpd : Outport  Port=32  VectorParamsAs1DForOutWhenUnconnected=off
  GenPwrElec : Outport  Port=33  VectorParamsAs1DForOutWhenUnconnected=off
  GenPwrMech : Outport  Port=34  VectorParamsAs1DForOutWhenUnconnected=off
  BMS_Sensors : Outport  Port=35
  wires:
  PtCtrl/1 -> Bus Selector1/1
  OpCmds/1 -> Bus Selector5/1
  VehPlnt/1 -> Bus Selector4/1, Bus Selector2/1
  Unit Conversion6/1 -> Rate Transition8/1
  Unit Conversion1/1 -> Rate Transition3/1
  Unit Conversion14/1 -> Rate Transition16/1
  Unit Conversion12/1 -> Rate Transition14/1
  Unit Conversion2/1 -> Rate Transition4/1
  Unit Conversion13/1 -> Rate Transition15/1
  Unit Conversion7/1 -> Rate Transition9/1
  Unit Conversion4/1 -> Rate Transition6/1
  Unit Conversion3/1 -> Rate Transition5/1
  Unit Conversion5/1 -> Rate Transition7/1
  Unit Conversion10/1 -> Rate Transition12/1
  Unit Conversion11/1 -> Rate Transition13/1
  Unit Conversion/1 -> Rate Transition2/1
  Unit Conversion9/1 -> Rate Transition11/1
  Unit Conversion8/1 -> Rate Transition10/1
  Unit Conversion15/1 -> Rate Transition18/1
  Env/1 -> Bus Selector3/1
  Unit Conversion17/1 -> Rate Transition20/1
  Unit Conversion16/1 -> Rate Transition19/1
  Unit Conversion18/1 -> Rate Transition17/1
  Bus Selector3/1 -> Rate Transition1/1  "<Baro>"
  Bus Selector4/1 -> Unit Conversion/1  "<EngSpd>"
  Bus Selector4/2 -> Unit Conversion1/1  "<Map>"
  Bus Selector4/3 -> Unit Conversion2/1  "<Mat>"
  Bus Selector4/4 -> Unit Conversion3/1  "<ThrPosPct>"
  Bus Selector4/5 -> Unit Conversion4/1  "<WgAreaPct>"
  Bus Selector4/6 -> Unit Conversion5/1  "<IntkCamPhase>"
  Bus Selector4/7 -> Unit Conversion6/1  "<ExhCamPhase>"
  Bus Selector4/8 -> Unit Conversion7/1  "<TurboRackPos>"
  Bus Selector4/9 -> Unit Conversion8/1  "<EgrVlvAreaPct>"
  Bus Selector4/10 -> Unit Conversion9/1  "<VarCompRatioPos>"
  Bus Selector4/11 -> Unit Conversion10/1  "<IntkVlvLift>"
  Bus Selector4/12 -> Unit Conversion11/1  "<VarIntkRunLen>"
  Bus Selector4/13 -> Unit Conversion12/1  "<Afr>"
  Bus Selector4/14 -> Unit Conversion13/1  "<IntkSwirlVlvPos>"
  Bus Selector4/15 -> Unit Conversion14/1  "<TurboSpd>"
  Bus Selector4/16 -> Unit Conversion18/1  "<Iat>"
  Bus Selector4/17 -> Unit Conversion15/1  "<Ect>"
  Bus Selector4/18 -> Unit Conversion16/1  "<EgrVlvDeltaPrs>"
  Bus Selector4/19 -> Unit Conversion17/1  "<EgrVlvInTemp>"
  Bus Selector5/1 -> Rate Transition21/1  "<Accel>"
  Bus Selector5/2 -> Rate Transition22/1  "<Decel>"
  Bus Selector5/3 -> Rate Transition23/1  "<IgSw>"
  Bus Selector2/1 -> Rate Transition24/1  "<VehSpdDriveTrain>"
  Bus Selector2/2 -> Rate Transition25/1  "<EngSpd>"
  Bus Selector2/3 -> Rate Transition26/1  "<EngCltchState>"
  Bus Selector2/4 -> Rate Transition27/1  "<BattSoc>"
  Bus Selector2/5 -> Rate Transition28/1  "<BattPwr>"
  Bus Selector2/6 -> Rate Transition29/1  "<BattCrnt>"
  Bus Selector2/7 -> Rate Transition30/1  "<EngCltchOutSpd>"
  Bus Selector2/8 -> Rate Transition31/1  "<MotSpd>"
  Bus Selector2/9 -> Rate Transition32/1  "<GenPwrElec>"
  Bus Selector2/10 -> Rate Transition33/1  "<GenPwrMech>"
  Bus Selector1/1 -> Rate Transition/1  "<EngineTrqCmd>"
  Rate Transition10/1 -> EgrVlvAreaPct/1
  Rate Transition1/1 -> AmbPrs/1
  Rate Transition12/1 -> IntkVlvLift/1
  Rate Transition11/1 -> VarCompRatioPos/1
  Rate Transition13/1 -> VarIntkRunLen/1
  Rate Transition15/1 -> IntkSwirlVlvPos/1
  Rate Transition14/1 -> Afr/1
  Rate Transition16/1 -> TurboSpd/1
  Rate Transition19/1 -> EgrDeltaPrs/1
  Rate Transition17/1 -> Iat/1
  Rate Transition18/1 -> Ect/1
  Rate Transition2/1 -> EngSpd/1
  Rate Transition3/1 -> Map/1
  Rate Transition20/1 -> EgrInTemp/1
  Rate Transition4/1 -> Mat/1
  Rate Transition5/1 -> ThrPosPct/1
  Rate Transition6/1 -> WgAreaPct/1
  Rate Transition9/1 -> TurboRackPos/1
  Rate Transition7/1 -> IntkCamPhase/1
  Rate Transition8/1 -> ExhCamPhase/1
  Rate Transition/1 -> TrqCmd/1
  Rate Transition21/1 -> AccCmd/1
  Rate Transition22/1 -> DecCmd/1
  Rate Transition23/1 -> IgSw/1
  Rate Transition24/1 -> VehSpdFdbk/1
  Rate Transition25/1 -> EngSpdFdbk/1
  Rate Transition26/1 -> EngCltchState/1
  Rate Transition27/1 -> BattSoc/1
  Rate Transition28/1 -> BattPwr/1
  Rate Transition30/1 -> EngCltchOutSpd/1
  Rate Transition29/1 -> BattCrnt/1
  Rate Transition31/1 -> MotSpd/1
  Rate Transition32/1 -> GenPwrElec/1
  Rate Transition33/1 -> GenPwrMech/1
  Bus Selector2/11 -> Rate Transition34/1  "<BMS_Sensors>"
  Rate Transition34/1 -> BMS_Sensors/1

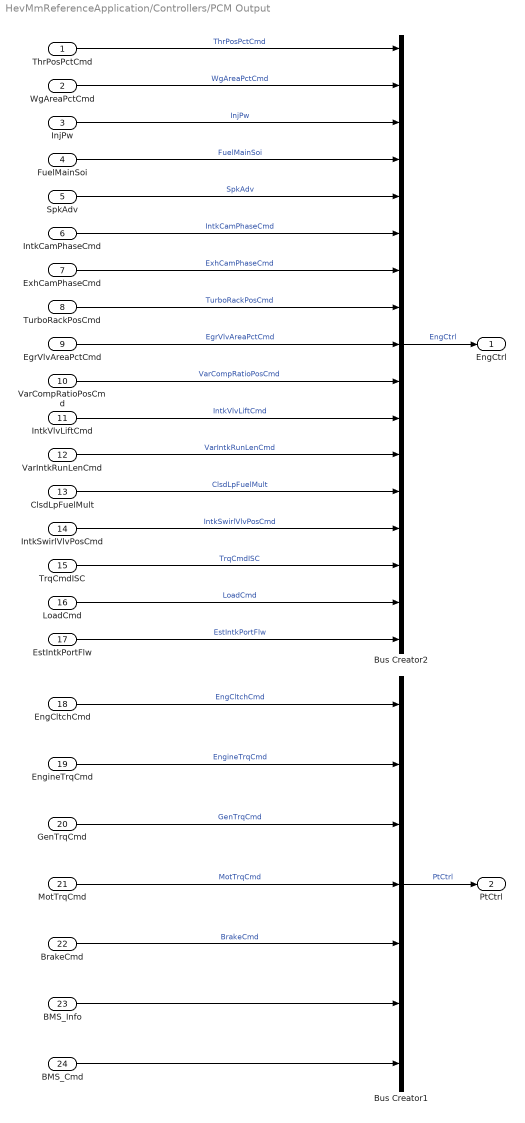
== system HevMmReferenceApplication/Controllers/PCM Output ==
  ThrPosPctCmd : Inport
  WgAreaPctCmd : Inport  Port=2
  InjPw : Inport  Port=3
  FuelMainSoi : Inport  Port=4
  SpkAdv : Inport  Port=5
  IntkCamPhaseCmd : Inport  Port=6
  ExhCamPhaseCmd : Inport  Port=7
  TurboRackPosCmd : Inport  Port=8
  EgrVlvAreaPctCmd : Inport  Port=9
  VarCompRatioPosCmd : Inport  Port=10
  IntkVlvLiftCmd : Inport  Port=11
  VarIntkRunLenCmd : Inport  Port=12
  ClsdLpFuelMult : Inport  Port=13
  IntkSwirlVlvPosCmd : Inport  Port=14
  TrqCmdISC : Inport  Port=15
  LoadCmd : Inport  Port=16
  EstIntkPortFlw : Inport  Port=17
  EngCltchCmd : Inport  Port=18
  EngineTrqCmd : Inport  Port=19
  GenTrqCmd : Inport  Port=20
  MotTrqCmd : Inport  Port=21
  BrakeCmd : Inport  Port=22
  BMS_Info : Inport  Port=23
  BMS_Cmd : Inport  Port=24
  Bus Creator1 : BusCreator  Inputs=7
  Bus Creator2 : BusCreator  Inputs=17
  EngCtrl : Outport  VectorParamsAs1DForOutWhenUnconnected=off
  PtCtrl : Outport  Port=2  VectorParamsAs1DForOutWhenUnconnected=off
  wires:
  BrakeCmd/1 -> Bus Creator1/5  "BrakeCmd"
  Bus Creator1/1 -> PtCtrl/1  "PtCtrl"
  EngCltchCmd/1 -> Bus Creator1/1  "EngCltchCmd"
  EngineTrqCmd/1 -> Bus Creator1/2  "EngineTrqCmd"
  GenTrqCmd/1 -> Bus Creator1/3  "GenTrqCmd"
  MotTrqCmd/1 -> Bus Creator1/4  "MotTrqCmd"
  Bus Creator2/1 -> EngCtrl/1  "EngCtrl"
  LoadCmd/1 -> Bus Creator2/16  "LoadCmd"
  TurboRackPosCmd/1 -> Bus Creator2/8  "TurboRackPosCmd"
  InjPw/1 -> Bus Creator2/3  "InjPw"
  IntkSwirlVlvPosCmd/1 -> Bus Creator2/14  "IntkSwirlVlvPosCmd"
  FuelMainSoi/1 -> Bus Creator2/4  "FuelMainSoi"
  ThrPosPctCmd/1 -> Bus Creator2/1  "ThrPosPctCmd"
  VarIntkRunLenCmd/1 -> Bus Creator2/12  "VarIntkRunLenCmd"
  TrqCmdISC/1 -> Bus Creator2/15  "TrqCmdISC"
  IntkCamPhaseCmd/1 -> Bus Creator2/6  "IntkCamPhaseCmd"
  EgrVlvAreaPctCmd/1 -> Bus Creator2/9  "EgrVlvAreaPctCmd"
  WgAreaPctCmd/1 -> Bus Creator2/2  "WgAreaPctCmd"
  SpkAdv/1 -> Bus Creator2/5  "SpkAdv"
  EstIntkPortFlw/1 -> Bus Creator2/17  "EstIntkPortFlw"
  ClsdLpFuelMult/1 -> Bus Creator2/13  "ClsdLpFuelMult"
  VarCompRatioPosCmd/1 -> Bus Creator2/10  "VarCompRatioPosCmd"
  ExhCamPhaseCmd/1 -> Bus Creator2/7  "ExhCamPhaseCmd"
  IntkVlvLiftCmd/1 -> Bus Creator2/11  "IntkVlvLiftCmd"
  BMS_Info/1 -> Bus Creator1/6
  BMS_Cmd/1 -> Bus Creator1/7

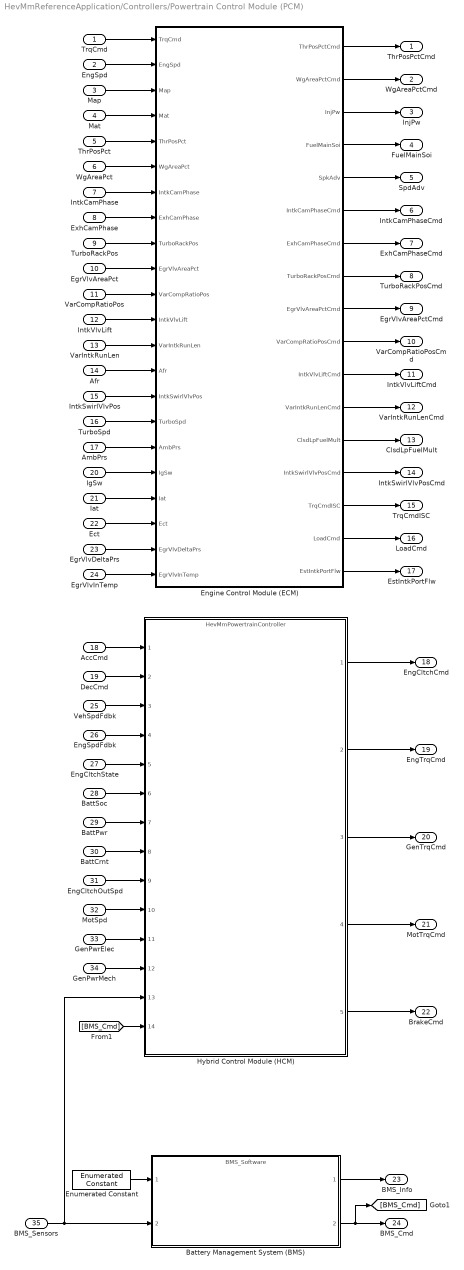
== system HevMmReferenceApplication/Controllers/Powertrain Control Module (PCM) ==
  TrqCmd : Inport
  EngSpd : Inport  Port=2
  Map : Inport  Port=3
  Mat : Inport  Port=4
  ThrPosPct : Inport  Port=5
  WgAreaPct : Inport  Port=6
  IntkCamPhase : Inport  Port=7
  ExhCamPhase : Inport  Port=8
  TurboRackPos : Inport  Port=9
  EgrVlvAreaPct : Inport  Port=10
  VarCompRatioPos : Inport  Port=11
  IntkVlvLift : Inport  Port=12
  VarIntkRunLen : Inport  Port=13
  Afr : Inport  Port=14
  IntkSwirlVlvPos : Inport  Port=15
  TurboSpd : Inport  Port=16
  AmbPrs : Inport  Port=17
  AccCmd : Inport  Port=18
  DecCmd : Inport  Port=19
  IgSw : Inport  Port=20
  Iat : Inport  Port=21
  Ect : Inport  Port=22
  EgrVlvDeltaPrs : Inport  Port=23
  EgrVlvInTemp : Inport  Port=24
  VehSpdFdbk : Inport  Port=25
  EngSpdFdbk : Inport  Port=26
  EngCltchState : Inport  Port=27
  BattSoc : Inport  Port=28
  BattPwr : Inport  Port=29
  BattCrnt : Inport  Port=30
  EngCltchOutSpd : Inport  Port=31
  MotSpd : Inport  Port=32
  GenPwrElec : Inport  Port=33
  GenPwrMech : Inport  Port=34
  BMS_Sensors : Inport  Port=35  LockScale=on
  Battery Management System (BMS) : ModelReference  ModelNameDialog=BMS_Software.slx  ModelReferenceVersion=3.6
  Engine Control Module (ECM) : Subsystem  Variant=on  VariantControlMode=label  LabelModeActiveChoice=SiEngineController
  Enumerated Constant : simulink/Sources/Enumerated Constant  OutDataTypeStr=Enum: SRE  Value=SRE.Charging  SampleTime=inf
  Hybrid Control Module (HCM) : ModelReference  ModelNameDialog=HevMmPowertrainController.slx  ModelReferenceVersion=5.37
  ThrPosPctCmd : Outport  VectorParamsAs1DForOutWhenUnconnected=off
  WgAreaPctCmd : Outport  Port=2  VectorParamsAs1DForOutWhenUnconnected=off
  InjPw : Outport  Port=3  VectorParamsAs1DForOutWhenUnconnected=off
  FuelMainSoi : Outport  Port=4  VectorParamsAs1DForOutWhenUnconnected=off
  SpdAdv : Outport  Port=5  VectorParamsAs1DForOutWhenUnconnected=off
  IntkCamPhaseCmd : Outport  Port=6  VectorParamsAs1DForOutWhenUnconnected=off
  ExhCamPhaseCmd : Outport  Port=7  VectorParamsAs1DForOutWhenUnconnected=off
  TurboRackPosCmd : Outport  Port=8  VectorParamsAs1DForOutWhenUnconnected=off
  EgrVlvAreaPctCmd : Outport  Port=9  VectorParamsAs1DForOutWhenUnconnected=off
  VarCompRatioPosCmd : Outport  Port=10  VectorParamsAs1DForOutWhenUnconnected=off
  IntkVlvLiftCmd : Outport  Port=11  VectorParamsAs1DForOutWhenUnconnected=off
  VarIntkRunLenCmd : Outport  Port=12  VectorParamsAs1DForOutWhenUnconnected=off
  ClsdLpFuelMult : Outport  Port=13  VectorParamsAs1DForOutWhenUnconnected=off
  IntkSwirlVlvPosCmd : Outport  Port=14  VectorParamsAs1DForOutWhenUnconnected=off
  TrqCmdISC : Outport  Port=15  VectorParamsAs1DForOutWhenUnconnected=off
  LoadCmd : Outport  Port=16  VectorParamsAs1DForOutWhenUnconnected=off
  EstIntkPortFlw : Outport  Port=17  VectorParamsAs1DForOutWhenUnconnected=off
  EngCltchCmd : Outport  Port=18  VectorParamsAs1DForOutWhenUnconnected=off
  EngTrqCmd : Outport  Port=19  VectorParamsAs1DForOutWhenUnconnected=off
  GenTrqCmd : Outport  Port=20  VectorParamsAs1DForOutWhenUnconnected=off
  MotTrqCmd : Outport  Port=21  VectorParamsAs1DForOutWhenUnconnected=off
  BrakeCmd : Outport  Port=22  VectorParamsAs1DForOutWhenUnconnected=off
  BMS_Info : Outport  Port=23
  BMS_Cmd : Outport  Port=24
  wires:
  BattSoc/1 -> Hybrid Control Module (HCM)/6
  GenPwrMech/1 -> Hybrid Control Module (HCM)/12
  VehSpdFdbk/1 -> Hybrid Control Module (HCM)/3
  Hybrid Control Module (HCM)/2 -> EngTrqCmd/1
  Hybrid Control Module (HCM)/5 -> BrakeCmd/1
  Hybrid Control Module (HCM)/3 -> GenTrqCmd/1
  MotSpd/1 -> Hybrid Control Module (HCM)/10
  GenPwrElec/1 -> Hybrid Control Module (HCM)/11
  EngCltchOutSpd/1 -> Hybrid Control Module (HCM)/9
  Hybrid Control Module (HCM)/4 -> MotTrqCmd/1
  Hybrid Control Module (HCM)/1 -> EngCltchCmd/1
  EngCltchState/1 -> Hybrid Control Module (HCM)/5
  BattPwr/1 -> Hybrid Control Module (HCM)/7
  BattCrnt/1 -> Hybrid Control Module (HCM)/8
  AccCmd/1 -> Hybrid Control Module (HCM)/1
  EngSpdFdbk/1 -> Hybrid Control Module (HCM)/4
  DecCmd/1 -> Hybrid Control Module (HCM)/2
  VarCompRatioPos/1 -> Engine Control Module (ECM)/11(VarCompRatioPos)
  IntkVlvLift/1 -> Engine Control Module (ECM)/12(IntkVlvLift)
  VarIntkRunLen/1 -> Engine Control Module (ECM)/13(VarIntkRunLen)
  Afr/1 -> Engine Control Module (ECM)/14(Afr)
  IntkSwirlVlvPos/1 -> Engine Control Module (ECM)/15(IntkSwirlVlvPos)
  WgAreaPct/1 -> Engine Control Module (ECM)/6(WgAreaPct)
  ThrPosPct/1 -> Engine Control Module (ECM)/5(ThrPosPct)
  EgrVlvAreaPct/1 -> Engine Control Module (ECM)/10(EgrVlvAreaPct)
  TurboRackPos/1 -> Engine Control Module (ECM)/9(TurboRackPos)
  Mat/1 -> Engine Control Module (ECM)/4(Mat)
  Map/1 -> Engine Control Module (ECM)/3(Map)
  EngSpd/1 -> Engine Control Module (ECM)/2(EngSpd)
  TrqCmd/1 -> Engine Control Module (ECM)/1(TrqCmd)
  AmbPrs/1 -> Engine Control Module (ECM)/17(AmbPrs)
  TurboSpd/1 -> Engine Control Module (ECM)/16(TurboSpd)
  ExhCamPhase/1 -> Engine Control Module (ECM)/8(ExhCamPhase)
  IntkCamPhase/1 -> Engine Control Module (ECM)/7(IntkCamPhase)
  IgSw/1 -> Engine Control Module (ECM)/18(IgSw)
  Ect/1 -> Engine Control Module (ECM)/20(Ect)
  Engine Control Module (ECM)/1(ThrPosPctCmd) -> ThrPosPctCmd/1
  Engine Control Module (ECM)/2(WgAreaPctCmd) -> WgAreaPctCmd/1
  Engine Control Module (ECM)/3(InjPw) -> InjPw/1
  Engine Control Module (ECM)/4(FuelMainSoi) -> FuelMainSoi/1
  Engine Control Module (ECM)/5(SpkAdv) -> SpdAdv/1
  Engine Control Module (ECM)/6(IntkCamPhaseCmd) -> IntkCamPhaseCmd/1
  Engine Control Module (ECM)/7(ExhCamPhaseCmd) -> ExhCamPhaseCmd/1
  Engine Control Module (ECM)/8(TurboRackPosCmd) -> TurboRackPosCmd/1
  Engine Control Module (ECM)/9(EgrVlvAreaPctCmd) -> EgrVlvAreaPctCmd/1
  Engine Control Module (ECM)/10(VarCompRatioPosCmd) -> VarCompRatioPosCmd/1
  Engine Control Module (ECM)/11(IntkVlvLiftCmd) -> IntkVlvLiftCmd/1
  Engine Control Module (ECM)/12(VarIntkRunLenCmd) -> VarIntkRunLenCmd/1
  Engine Control Module (ECM)/13(ClsdLpFuelMult) -> ClsdLpFuelMult/1
  Engine Control Module (ECM)/14(IntkSwirlVlvPosCmd) -> IntkSwirlVlvPosCmd/1
  Engine Control Module (ECM)/15(TrqCmdISC) -> TrqCmdISC/1
  Engine Control Module (ECM)/16(LoadCmd) -> LoadCmd/1
  Engine Control Module (ECM)/17(EstIntkPortFlw) -> EstIntkPortFlw/1
  EgrVlvDeltaPrs/1 -> Engine Control Module (ECM)/21(EgrVlvDeltaPrs)
  EgrVlvInTemp/1 -> Engine Control Module (ECM)/22(EgrVlvInTemp)
  Iat/1 -> Engine Control Module (ECM)/19(Iat)
  Battery Management System (BMS)/1 -> BMS_Info/1
  BMS_Sensors/1 -> Hybrid Control Module (HCM)/13, Battery Management System (BMS)/2
  Battery Management System (BMS)/2 -> [BMS_Cmd], BMS_Cmd/1
  Enumerated Constant/1 -> Battery Management System (BMS)/1
  [BMS_Cmd] -> Hybrid Control Module (HCM)/14

== system HevMmReferenceApplication/Longitudinal Driver/Longitudinal Driver ==
  Vref : Inport
  Vfdbk : Inport  Port=2
  Bus Creator1 : BusCreator  Inputs=2
  Bus Selector : BusSelector  OutputSignals=Veh.VehSpdDriveTrain
  Constant : Constant  Value=false
  Data Type Conversion : DataTypeConversion  OutDataTypeStr=boolean
  Ground : Ground
  Ignition Switch Profile : Subsystem  Tag=STV Subsys  LoadFcn=sigbuilder_block('load');  StartFcn=sigbuilder_block('start');  StopFcn=sigbuilder_block('stop');  ClipboardFcn=sigbuilder_block('clipboard');  mask(Sigbuilder block){tuvar=[0:10]}
      mask help: Simulink:masks:SigbuilderBlock_MD
      mask init:
      | if ~strcmp(get_param(bdroot(gcbh),'SimulationStatus'),'stopped') tuvar = sigbuilder_block('maskInit'); end
      settings: CopyFcn=sigbuilder_block('copy');  DeleteFcn=sigbuilder_block('delete');  ModelCloseFcn=sigbuilder_block('modelClose');  PreSaveFcn=sigbuilder_block('preSave');  PauseFcn=sigbuilder_block('pause');  ContinueFcn=sigbuilder_block('continue');  NameChangeFcn=sigbuilder_block('namechange');  OpenFcn=sigbuilder_block('open',[595.8 176.4 550.8 322.2 ]);  CloseFcn=sigbuilder_block('close');
      mask Display: plot(0, 0, 100, 100,[2, 2, 32, 32, 2], [68, 8, 8, 68, 68],[32, 2], [38, 38], [32, 19, 2],[53, 60, 44], [32, 17, 17, 2],[16, 16, 31, 31]);txt = getActiveGroup(gcbh);text(2, 100, txt,'verticalAlignment', 'top');
  Longitudinal Driver Model : autolibshared/Longitudinal Driver  extAccelOvr=off  extDecelOvr=off  extAccelHld=off  extDecelHld=off  extAccelZero=off  extDecelZero=off  cntrlType=PI  shftType=None  velUnits=m/s  gearOut=off  Kp=1.3  Ki=0.05  Kff=0  Kg=0  VehVelVec=[0 100]  KffVec=[.1 .1]  KpVec=[10 10]  KiVec=[5 5]  KgVec=[0 0]  m=1500  Kpt=10000  tau=0.12  L=4  aR=30.3/3875  bR=0.21290*4.44822/0.44704  cR=0.36  g=9.81  vnom=5  Kaw=1  tauerr=0.01  tauPt=2  GearInit=0  tShift=.1  pdlVec=[0.1 0.4 0.5 0.9]  upShftTbl=[-1 12.9375 26.4375 39.9375 51.18749999999999 62.4375 72.84375 83.25;-1 16.3125 29.8125 43.3125 54.5624 65.8125 76.78125 87.75;-1 19.6875 33.1875 46.68749999999999 57.9375 69.1875 80.71875 92.25;-1 33 52.5 77.25 100.5 138.75 161.875 185]  dwnShftTbl=[1 9.5625 23.0625 36.5625 47.8125 59.0625 68.90625 78.75;1 12.9375 26.4375 39.9375 51.18749999999999 62.4375 72.84375 83.25;1 16.3125 29.8125 43.3125 54.562499 65.8125 76.78125 87.75;1 19.6875 33.1875 46.68749999999999 57.9375 69.1875 80.71875 92.25]  tClutch=.5  tRev=.5  tPark=120  aMode=1  UpGearVec="[0  1  2  3  4  5  6  7]"  DownGearVec="[1  2  3  4  5  6  7  8]"
      settings: SourceProductBaseCode=PW,DR,MT,UV,VE
  Manual Switch : ManualSwitch
  Terminator : Terminator
  Terminator1 : Terminator
  OpCmds : Outport  VectorParamsAs1DForOutWhenUnconnected=off
  wires:
  Vfdbk/1 -> Bus Selector/1
  Ground/1 -> Longitudinal Driver Model/3
  Bus Selector/1 -> Longitudinal Driver Model/2  "<VehSpdDriveTrain>"
  Bus Creator1/1 -> OpCmds/1
  Longitudinal Driver Model/1 -> Bus Creator1/1  "Info"
  Longitudinal Driver Model/2 -> Terminator/1  "Acc"
  Ignition Switch Profile/1(IGSW) -> Data Type Conversion/1
  Data Type Conversion/1 -> Manual Switch/2
  Manual Switch/1 -> Bus Creator1/2  "IgSw"
  Vref/1 -> Longitudinal Driver Model/1  "xdotref"
  Longitudinal Driver Model/3 -> Terminator1/1  "Dec"
  Constant/1 -> Manual Switch/1

== system HevMmReferenceApplication/Longitudinal Driver/Open Loop ==
  note: This subsystem is provided to disable the driver subsystem and expose the driver interface.
      |
      | The interface can:
      | - be connected with dashboard UI blocks or 3rd party hardware
      | - provide application specific pre-programmed event or time based signals
      | - be driven by recorded operator signals for tuning, troubleshooting and model validation
  Bus Creator1 : BusCreator  Inputs=2
  Bus Creator2 : BusCreator  Inputs=8
  Constant : Constant  Value=false
  Constant{1..4} (4 alike) : Constant  Value=0
  Data Type Conversion : DataTypeConversion  OutDataTypeStr=boolean
  Ground{,1..3} (4 alike) : Ground
  Ignition Switch Profile : Subsystem  Tag=STV Subsys  LoadFcn=sigbuilder_block('load');  StartFcn=sigbuilder_block('start');  StopFcn=sigbuilder_block('stop');  ClipboardFcn=sigbuilder_block('clipboard');  mask(Sigbuilder block){tuvar=[0:10]}
      mask help: Simulink:masks:SigbuilderBlock_MD
      mask init:
      | if ~strcmp(get_param(bdroot(gcbh),'SimulationStatus'),'stopped') tuvar = sigbuilder_block('maskInit'); end
      settings: CopyFcn=sigbuilder_block('copy');  DeleteFcn=sigbuilder_block('delete');  ModelCloseFcn=sigbuilder_block('modelClose');  PreSaveFcn=sigbuilder_block('preSave');  PauseFcn=sigbuilder_block('pause');  ContinueFcn=sigbuilder_block('continue');  NameChangeFcn=sigbuilder_block('namechange');  OpenFcn=sigbuilder_block('open',[595.8 176.4 550.8 322.2 ]);  CloseFcn=sigbuilder_block('close');
      mask Display: plot(0, 0, 100, 100,[2, 2, 32, 32, 2], [68, 8, 8, 68, 68],[32, 2], [38, 38], [32, 19, 2],[53, 60, 44], [32, 17, 17, 2],[16, 16, 31, 31]);txt = getActiveGroup(gcbh);text(2, 100, txt,'verticalAlignment', 'top');
  Manual Switch : ManualSwitch
  OpCmds : Outport  VectorParamsAs1DForOutWhenUnconnected=off
  wires:
  Constant4/1 -> Bus Creator2/4  "Clutch"
  Ground/1 -> Bus Creator2/5  "Err"
  Constant2/1 -> Bus Creator2/2  "Decel"
  Constant3/1 -> Bus Creator2/3  "Gear"
  Constant1/1 -> Bus Creator2/1  "Accel"
  Ground2/1 -> Bus Creator2/7  "ErrMax"
  Bus Creator2/1 -> Bus Creator1/1  "Info"
  Ground1/1 -> Bus Creator2/6  "ErrSqrSum"
  Ground3/1 -> Bus Creator2/8  "ErrMin"
  Ignition Switch Profile/1(IGSW) -> Data Type Conversion/1
  Manual Switch/1 -> Bus Creator1/2  "IgSw"
  Bus Creator1/1 -> OpCmds/1
  Constant/1 -> Manual Switch/1
  Data Type Conversion/1 -> Manual Switch/2

== system HevMmReferenceApplication/Longitudinal Driver/PID ==
  Vref : Inport
  Vfdbk : Inport  Port=2
  Bus Creator1 : BusCreator  Inputs=2
  Bus Selector : BusSelector  OutputSignals=Veh.VehSpdDriveTrain
  Constant : Constant  Value=false
  Data Type Conversion : DataTypeConversion  OutDataTypeStr=boolean
  Driver Model : Subsystem
  Ground : Ground
  Ignition Switch Profile : Subsystem  Tag=STV Subsys  LoadFcn=sigbuilder_block('load');  StartFcn=sigbuilder_block('start');  StopFcn=sigbuilder_block('stop');  ClipboardFcn=sigbuilder_block('clipboard');  mask(Sigbuilder block){tuvar=[0:10]}
      mask help: Simulink:masks:SigbuilderBlock_MD
      mask init:
      | if ~strcmp(get_param(bdroot(gcbh),'SimulationStatus'),'stopped') tuvar = sigbuilder_block('maskInit'); end
      settings: CopyFcn=sigbuilder_block('copy');  DeleteFcn=sigbuilder_block('delete');  ModelCloseFcn=sigbuilder_block('modelClose');  PreSaveFcn=sigbuilder_block('preSave');  PauseFcn=sigbuilder_block('pause');  ContinueFcn=sigbuilder_block('continue');  NameChangeFcn=sigbuilder_block('namechange');  OpenFcn=sigbuilder_block('open',[595.8 176.4 550.8 322.2 ]);  CloseFcn=sigbuilder_block('close');
      mask Display: plot(0, 0, 100, 100,[2, 2, 32, 32, 2], [68, 8, 8, 68, 68],[32, 2], [38, 38], [32, 19, 2],[53, 60, 44], [32, 17, 17, 2],[16, 16, 31, 31]);txt = getActiveGroup(gcbh);text(2, 100, txt,'verticalAlignment', 'top');
  Manual Switch : ManualSwitch
  Terminator : Terminator
  Terminator1 : Terminator
  OpCmds : Outport  VectorParamsAs1DForOutWhenUnconnected=off
  wires:
  Vfdbk/1 -> Bus Selector/1
  Vref/1 -> Driver Model/1(Vref)
  Bus Selector/1 -> Driver Model/2(VelFdbk)  "<VehSpdDriveTrain>"
  Ground/1 -> Driver Model/3(Grade)
  Driver Model/2(AccelCmd) -> Terminator/1  "Acc"
  Ignition Switch Profile/1(IGSW) -> Data Type Conversion/1
  Manual Switch/1 -> Bus Creator1/2  "IgSw"
  Driver Model/3(DecelCmd) -> Terminator1/1  "Dec"
  Driver Model/1(Info) -> Bus Creator1/1  "Info"
  Bus Creator1/1 -> OpCmds/1
  Data Type Conversion/1 -> Manual Switch/2
  Constant/1 -> Manual Switch/1

== system HevMmReferenceApplication/Passenger Car/Drivetrain Output ==
  VehSpd : Inport
  "EngSpd " : Inport  Port=2
  EngCltchState : Inport  Port=3
  GenSpd : Inport  Port=4
  MotSpd : Inport  Port=5
  EngCltchOutSpd : Inport  Port=6
  Bus Creator1 : BusCreator  Inputs=5
  Bus Creator3 : BusCreator  Inputs=1
  VehFdbk : Outport  VectorParamsAs1DForOutWhenUnconnected=off
  EngFdbk : Outport  Port=2  VectorParamsAs1DForOutWhenUnconnected=off
  wires:
  Bus Creator1/1 -> VehFdbk/1  "VehFdbk"
  VehSpd/1 -> Bus Creator1/1
  "EngSpd "/1 -> Bus Creator3/1  "EngSpd"
  Bus Creator3/1 -> EngFdbk/1  "EngFdbk"
  EngCltchState/1 -> Bus Creator1/2  "EngCltchState"
  GenSpd/1 -> Bus Creator1/3  "GenSpd"
  MotSpd/1 -> Bus Creator1/4  "MotSpd"
  EngCltchOutSpd/1 -> Bus Creator1/5  "EngCltchOutSpd"
